simulink model "UDE"  (R2020a)
settings: Solver=ode4  StartTime=0.0  StopTime=tstop  FixedStep=tstep  RelTol=1e-3
values from neighbouring files (symbols this model uses):
  eic = xic - xmic    [data.m]
  K = place(F_n, G_n, eig(F_m))    [data.m]
  Ts = 0.01    [data.m]
  udic = (-Ts/T)*pinv(G_n)*eic    [data.m]
  xic = [pi/6; -pi/6]    [data.m]
  xmic = [-pi/6; -pi/6]    [data.m]
settings Model: Creator=Ram Padmanabhan  LastModifiedBy=Ram Padmanabhan
settings DataIOCC: SaveOutput=off  SignalLogging=off  DSMLogging=off  SaveTime=off  ReturnWorkspaceOutputs=off

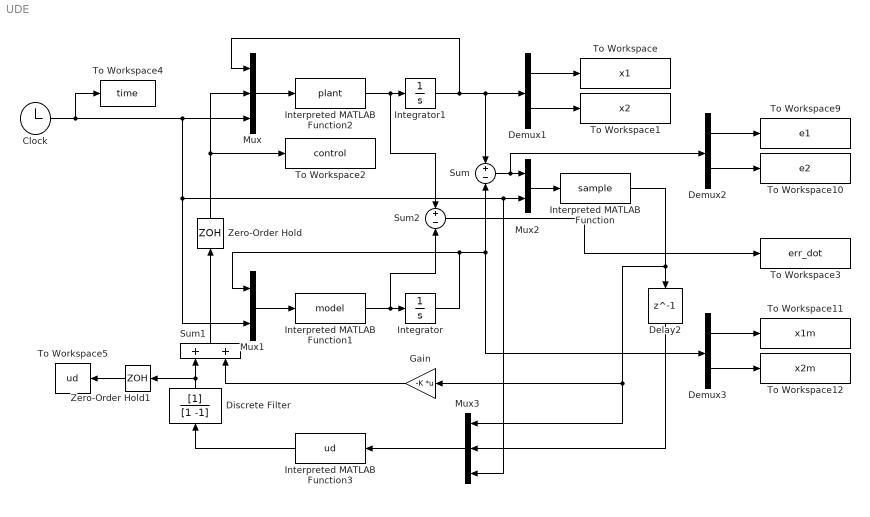
== system UDE ==
  Clock : Clock
  Delay2 : Delay  DelayLength=1  InitialCondition=eic  SampleTime=Ts
  Demux1 : Demux  Outputs=2
  Demux2 : Demux  Outputs=2
  Demux3 : Demux  Outputs=2
  Discrete Filter : DiscreteFilter  Denominator=[1 -1]  InitialStates=udic  SampleTime=Ts
  Gain : Gain  Gain=-K  Multiplication=Matrix(K*u)
  Integrator : Integrator  InitialCondition=xmic
  Integrator1 : Integrator  InitialCondition=xic
  Interpreted MATLAB Function : MATLABFcn  MATLABFcn=sample  OutputDimensions=2
  Interpreted MATLAB Function1 : MATLABFcn  MATLABFcn=model  OutputDimensions=2
  Interpreted MATLAB Function2 : MATLABFcn  MATLABFcn=plant  OutputDimensions=2
  Interpreted MATLAB Function3 : MATLABFcn  MATLABFcn=ud  OutputDimensions=1
  Mux : Mux  Inputs=3
  Mux1 : Mux  Inputs=2
  Mux2 : Mux  Inputs=2
  Mux3 : Mux  Inputs=3
  Sum : Sum  Inputs=+-
  Sum1 : Sum
  Sum2 : Sum  Inputs=+-
  To Workspace : ToWorkspace  VariableName=x1  SampleTime=-1
  To Workspace1 : ToWorkspace  VariableName=x2  SampleTime=-1
  To Workspace10 : ToWorkspace  VariableName=e2  SampleTime=-1
  To Workspace11 : ToWorkspace  VariableName=x1m  SampleTime=-1
  To Workspace12 : ToWorkspace  VariableName=x2m  SampleTime=-1
  To Workspace2 : ToWorkspace  VariableName=control  SampleTime=-1
  To Workspace3 : ToWorkspace  VariableName=err_dot  SampleTime=-1
  To Workspace4 : ToWorkspace  VariableName=time  SampleTime=-1
  To Workspace5 : ToWorkspace  VariableName=ud  SampleTime=-1
  To Workspace9 : ToWorkspace  VariableName=e1  SampleTime=-1
  Zero-Order Hold : ZeroOrderHold  SampleTime=Ts
  Zero-Order Hold1 : ZeroOrderHold  SampleTime=Ts
  wires:
  Interpreted MATLAB Function1/1 -> Sum2/2, Integrator/1
  Mux/1 -> Interpreted MATLAB Function2/1
  Integrator1/1 -> Sum/1, Demux1/1, Mux/1
  Integrator/1 -> Demux3/1, Sum/2, Mux1/1
  Mux1/1 -> Interpreted MATLAB Function1/1
  Clock/1 -> Mux3/3, Mux2/2, Mux1/2, Mux/3, To Workspace4/1
  Interpreted MATLAB Function2/1 -> Sum2/1, Integrator1/1
  Zero-Order Hold/1 -> To Workspace2/1, Mux/2
  Sum/1 -> Demux2/1, Mux2/1
  Mux2/1 -> Interpreted MATLAB Function/1
  Gain/1 -> Sum1/2
  Delay2/1 -> Mux3/2
  Interpreted MATLAB Function3/1 -> Discrete Filter/1
  Mux3/1 -> Interpreted MATLAB Function3/1
  Sum1/1 -> Zero-Order Hold/1
  Demux1/1 -> To Workspace/1
  Demux1/2 -> To Workspace1/1
  Demux2/1 -> To Workspace9/1
  Interpreted MATLAB Function/1 -> Delay2/1, Mux3/1, Gain/1
  Demux2/2 -> To Workspace10/1
  Demux3/1 -> To Workspace11/1
  Demux3/2 -> To Workspace12/1
  Zero-Order Hold1/1 -> To Workspace5/1
  Discrete Filter/1 -> Sum1/1, Zero-Order Hold1/1
  Sum2/1 -> To Workspace3/1
